simulink model "simPID11_08_14"  (R2014a)
settings: Solver=ode4  StartTime=0.0  StopTime=600  FixedStep=1  RelTol=1e-3
undefined symbols (not defined in the file): sigbuilder_block
settings Model: Creator=Cristian  LastModifiedBy=Cristian
settings SolverCC: MaxConsecutiveMinStep=0.1

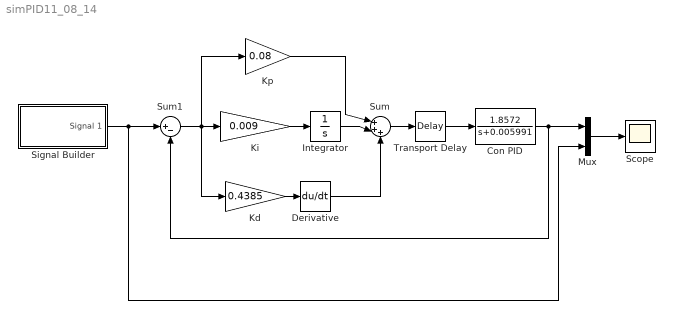
== system simPID11_08_14 ==
  Con PID : TransferFcn  Numerator=[1.8572]  Denominator=[1 0.005991]
  Derivative : Derivative
  Integrator : Integrator
  Kd : Gain  Gain=0.4385
  Ki : Gain  Gain=0.009
  Kp : Gain  Gain=0.08
  Mux : Mux  Inputs=2
  Scope : Scope
      settings: ShowLegends=on
  Signal Builder : Subsystem  Tag=STV Subsys  LoadFcn=sigbuilder_block('load');  StartFcn=sigbuilder_block('start');  StopFcn=sigbuilder_block('stop');  ClipboardFcn=sigbuilder_block('clipboard');  mask(Sigbuilder block){}
      mask help: Simulink:masks:SigbuilderBlock_MD
      mask init:
      | if ~strcmp(get_param(bdroot(gcbh),'SimulationStatus'),'stopped') tuvar = sigbuilder_block('maskInit'); end
      settings: CopyFcn=sigbuilder_block('copy');  DeleteFcn=sigbuilder_block('delete');  ModelCloseFcn=sigbuilder_block('modelClose');  PreSaveFcn=sigbuilder_block('preSave');  PauseFcn=sigbuilder_block('pause');  ContinueFcn=sigbuilder_block('continue');  NameChangeFcn=sigbuilder_block('namechange');  OpenFcn=sigbuilder_block('open',[138 66.75 550.5 394.5 ]);  CloseFcn=sigbuilder_block('close');
      mask Display: plot(0, 0, 100, 100,[2, 2, 32, 32, 2], [68, 8, 8, 68, 68],[32, 2], [38, 38], [32, 19, 2],[53, 60, 44], [32, 17, 17, 2],[16, 16, 31, 31]);txt = getActiveGroup(gcbh);text(2, 100, txt,'verticalAlignment', 'top');
  Sum : Sum  Inputs=|+++
  Sum1 : Sum  Inputs=|+-
  Transport Delay : TransportDelay  DelayTime=10
  wires:
  Kp/1 -> Sum/1
  Integrator/1 -> Sum/2
  Derivative/1 -> Sum/3
  Ki/1 -> Integrator/1
  Kd/1 -> Derivative/1
  Con PID/1 -> Sum1/2, Mux/1
  Signal Builder/1(Signal 1) -> Sum1/1, Mux/2
  Sum/1 -> Transport Delay/1
  Transport Delay/1 -> Con PID/1
  Mux/1 -> Scope/1
  Sum1/1 -> Ki/1, Kp/1, Kd/1

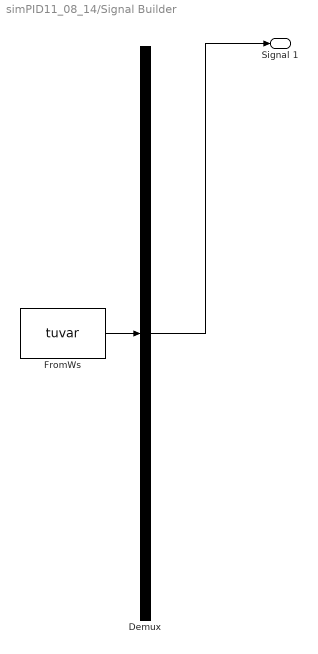
== system simPID11_08_14/Signal Builder ==
  Demux : Demux  Tag=STV Demux  Outputs=1
  FromWs : FromWorkspace  Tag=STV FromWs  VariableName=tuvar  SampleTime=0
      SigBuilderData=|
      | common.afterFinalStr = 'Extrapolate'
      | common.sampleTime = 0
      | dataSet.timeRange = [0 600]
      | dataSet.name = 'Group 1'
      | sbobj.Groups.Name = 'Group 1'
      | sbobj.Groups.Signals.Name = 'Signal 1'
      | sbobj.Groups.Signals.XData = [0 100 300 300 380 500 600]
      | sbobj.Groups.Signals.YData = [0 174 174 176 245 0 0]
      | sbobj.Groups.TimeRange = [0 600]
  Signal 1 : Outport  Tag=STV Outport
  wires:
  Demux/1 -> Signal 1/1
  FromWs/1 -> Demux/1
